simulink model "model"  (R2022b)
settings: Solver=VariableStepAuto  StartTime=0.0  StopTime=stopTime  MaxStep=0.01  RelTol=1e-3
values from neighbouring files (symbols this model uses):
  friction = friction(:,1:numSample)    [DataReading.m]    (also in DataSampling.m = random(frictionUniformDist, 1, numSample); SensitivityAnalysisConfig.m = 0.5; data.mat = [0.423870600502 0.414714985315 0.508364191084 0.585845302695)
  g = random(gDist, 1, 1)    [DataSampling.m]    (also in SensitivityAnalysisConfig.m = 9.8; data.mat = 9.78798650818)
  stopTime = 5    [DataReading.m]    (also in DataSampling.m; SensitivityAnalysisConfig.m)
  weight = weight(:,1:numSample)    [DataReading.m]    (also in DataSampling.m = random(weightDist, 1, numSample); SensitivityAnalysisConfig.m = 0.025; data.mat = [0.0249399431455 0.0249880813357 0.0249204436802 0.024988815)
libraries: simulink x1
settings Model: Creator=w.ar  LastModifiedBy=w.ar

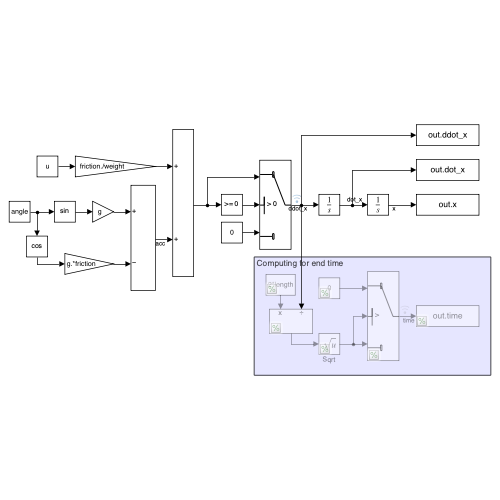
[thumbnail: Simulink's stored preview of the top-level diagram]
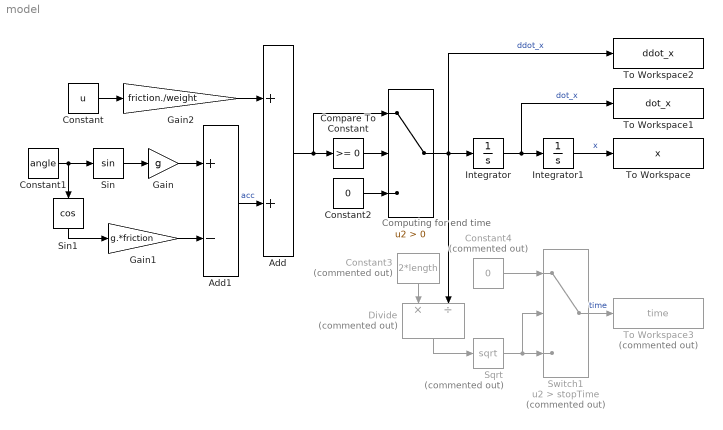
== system model ==
  note: Computing for end time
  Add : Sum
  Add1 : Sum  Inputs=+-
  Compare To Constant : simulink/Logic and Bit Operations/Compare To Constant  relop=>=  const=0  OutDataTypeStr=boolean
  Constant : Constant  Value=u
  Constant1 : Constant  Value=angle
  Constant2 : Constant  Value=0
  Constant3 : Constant  Commented=on  Value=2*length
  Constant4 : Constant  Commented=on  Value=0
  Divide : Product  Commented=on  Inputs=*/
  Gain : Gain  Gain=g
  Gain1 : Gain  Gain=g.*friction
  Gain2 : Gain  Gain=friction./weight
  Integrator : Integrator
  Integrator1 : Integrator  UpperSaturationLimit=length
  Sin : Trigonometry
  Sin1 : Trigonometry  Operator=cos
  Sqrt : Sqrt  Commented=on  IntermediateResultsDataTypeStr=double
  Switch : Switch  Criteria=u2 > Threshold  SaturateOnIntegerOverflow=off  InputSameDT=off
  Switch1 : Switch  Commented=on  Criteria=u2 > Threshold  Threshold=stopTime  SaturateOnIntegerOverflow=off  InputSameDT=off
  To Workspace : ToWorkspace  VariableName=x  SaveFormat=Timeseries  SampleTime=-1
  To Workspace1 : ToWorkspace  VariableName=dot_x  SaveFormat=Timeseries  SampleTime=-1
  To Workspace2 : ToWorkspace  VariableName=ddot_x  SaveFormat=Timeseries  SampleTime=-1
  To Workspace3 : ToWorkspace  Commented=on  VariableName=time  SaveFormat=Timeseries  SampleTime=-1
  wires:
  Gain1/1 -> Add1/2
  Constant2/1 -> Switch/3
  Sin1/1 -> Gain1/1
  Integrator/1 -> Integrator1/1, To Workspace1/1  "dot_x"
  Compare To Constant/1 -> Switch/2
  Sqrt/1 -> Switch1/3, Switch1/2
  Constant/1 -> Gain2/1
  Constant1/1 -> Sin/1, Sin1/1
  Gain/1 -> Add1/1
  Integrator1/1 -> To Workspace/1  "x"
  Gain2/1 -> Add/1
  Add/1 -> Switch/1, Compare To Constant/1
  Switch/1 -> Divide/2, Integrator/1, To Workspace2/1  "ddot_x"
  Add1/1 -> Add/2  "acc"
  Constant3/1 -> Divide/1
  Divide/1 -> Sqrt/1
  Sin/1 -> Gain/1
  Constant4/1 -> Switch1/1
  Switch1/1 -> To Workspace3/1  "time"
